simulink library "NxtrMath"  (R2013b)
settings: Solver=ode45  StartTime=0.0  StopTime=10.0  RelTol=1e-3
undefined symbols (not defined in the file or in its folder): ARCHGLBPRM_ONEOVER2PI_ULS_F32
libraries: FixdToFloat x2, FloatToFixd x2
settings Model: Creator=qzwc4r  LastModifiedBy=DZ1YRM

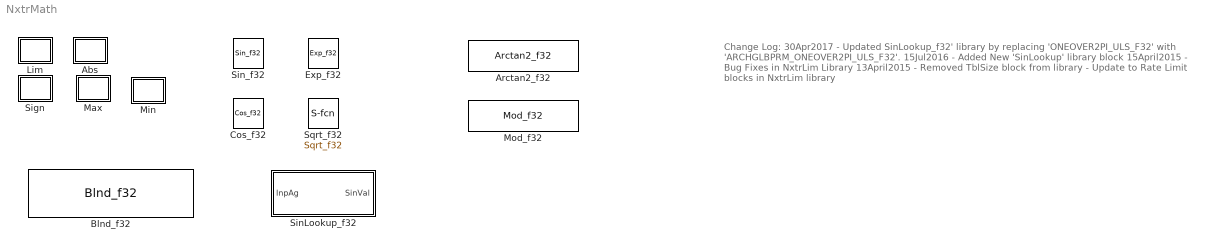
== system NxtrMath ==
  note: Change Log:
      |
      | 30Apr2017
      | - Updated SinLookup_f32' library by replacing 'ONEOVER2PI_ULS_F32' with 'ARCHGLBPRM_ONEOVER2PI_ULS_F32'.
      |
      | 15Jul2016
      | - Added New 'SinLookup' library block
      |
      |
      | 15April2015
      | - Bug Fixes in NxtrLim Library
      |
      |
      | 13April2015
      | - Removed TblSize block from library
      | - Update to Rate Limit blocks in NxtrLim library
  Abs : Subsystem
      settings: OpenFcn=NxtrAbslt
      mask Display: fprintf('|u|')
  Arctan2_f32 : S-Function  FunctionName=Arctan2_f32  EnableBusSupport=off  mask(Arctan2_f32){SFunctionSpec=single y1 = Arctan2_f32(single u1, single u2)}
      mask help:
      | This block allows you to call the legacy functions specified by the following Legacy Code Tool definition:
      | def.SFunctionName = 'Arctan2_f32';
      | def.OutputFcnSpec = 'single y1 = Arctan2_f32(single u1, single u2)';
      | def.HeaderFiles = {'NxtrMath.h', 'Std_Types.h', 'Platform_Types.h', 'Compiler.h', 'Compiler_Cfg.h'};
      | def.IncPaths = {'..\Nexteer_Utilities v3.0.0\SrcFiles'};
      settings: AttributesFormatString=%<MaskType>
      mask Help: <p>This block was generated automatically by the Legacy Code Tool. For detailed help on this tool, call<a href="matlab:legacy_code('help')"> legacy_code('help')</a>.</p>
      mask Display:
      | % time = (-0.4:0.001:0.4)
      | % plot(time+0.5,0.35*atan(20*pi*(time))+0.51)
      | fprintf('Arctan2')
      | port_label('input',1,'Numer')
      | port_label('input',2,'Denom')
      | port_label('Output',1,'Outp')
  Blnd_f32 : S-Function  FunctionName=Blnd_f32  EnableBusSupport=off  mask(Blnd_f32){SFunctionSpec=single y1 = Blnd_f32(single u1, single u2, single u3), Parameter3=on}
      mask prompts: Parameter3 "Show Figure"
      mask help:
      | This block allows you to call the legacy functions specified by the following Legacy Code Tool definition:
      | def.SFunctionName = 'Blnd_f32';
      | def.OutputFcnSpec = 'single y1 = Blnd_f32(single u1, single u2, single u3)';
      | def.HeaderFiles = {'NxtrMath.h', 'Std_Types.h', 'Platform_Types.h', 'Compiler.h', 'Compiler_Cfg.h'};
      | def.IncPaths = {'..\Nexteer_Utilities v3.0.0\SrcFiles'};
      settings: AttributesFormatString=%<Name>
      mask Help: <p>This block was generated automatically by the Legacy Code Tool. For detailed help on this tool, call<a href="matlab:legacy_code('help')"> legacy_code('help')</a>.</p>
      mask Display:
      | port_label('input',1,'Inp1')
      | port_label('input',2,'Inp2')
      | port_label('input',3,'Fac')
      | port_label('output',1,'Outp')
      | if Parameter3 == 1
      |     text(0.2,0.6,'\nInp1*(1 -Fac) ->|----|\n                        | + |-->\n    (Inp2*Fac) ->|----|')
      | end
  Cos_f32 : S-Function  FunctionName=Cos_f32  EnableBusSupport=off  mask(Cos_f32){SFunctionSpec=single y1 = Cos_f32(single u1)}
      mask help:
      | This block allows you to call the legacy functions specified by the following Legacy Code Tool definition:
      | def.SFunctionName = 'Cos_f32';
      | def.OutputFcnSpec = 'single y1 = Cos_f32(single u1)';
      | def.HeaderFiles = {'NxtrMath.h', 'Std_Types.h', 'Platform_Types.h', 'Compiler.h', 'Compiler_Cfg.h'};
      | def.IncPaths = {'..\Nexteer_Utilities v3.0.0\SrcFiles'};
      settings: AttributesFormatString=%<MaskType>
      mask Help: <p>This block was generated automatically by the Legacy Code Tool. For detailed help on this tool, call<a href="matlab:legacy_code('help')"> legacy_code('help')</a>.</p>
      mask Display: fprintf('Cos')
  Exp_f32 : S-Function  FunctionName=Exp_f32  EnableBusSupport=off  mask(Exp_f32){SFunctionSpec=single y1 = Exp_f32(single u1), ShowSpec=on}
      mask prompts: ShowSpec "Display function specification"
      mask help:
      | This block allows you to call the legacy functions specified by the following Legacy Code Tool definition:
      | def.SFunctionName = 'Exp_f32';
      | def.OutputFcnSpec = 'single y1 = Exp_f32(single u1)';
      | def.HeaderFiles = {'NxtrMath.h', 'Std_Types.h', 'Platform_Types.h', 'Compiler.h', 'Compiler_Cfg.h'};
      | def.IncPaths = {'..\Nexteer_Utilities v3.0.0\SrcFiles'};
      settings: AttributesFormatString=%<MaskType>
      mask Help: <p>This block was generated automatically by the Legacy Code Tool. For detailed help on this tool, call<a href="matlab:legacy_code('help')"> legacy_code('help')</a>.</p>
      mask Callback ShowSpec:
      | if strcmp(get_param(gcbh, 'ShowSpec'), 'on')
      |   set_param(gcbh, 'MaskDisplay', sprintf('fprintf(''%s'');', get_param(gcbh, 'SFunctionSpec')));
      | else
      |   set_param(gcbh, 'MaskDisplay', sprintf('fprintf(''%s'');', get_param(gcbh, 'FunctionName')));
      | end
      mask Display: fprintf('Exp');
  Lim : Subsystem
      settings: OpenFcn=NxtrLim
      mask Display: fprintf('Lim')
  Max : Subsystem
      settings: OpenFcn=NxtrMax
      mask Display: fprintf('Max')
  Min : Subsystem
      settings: OpenFcn=NxtrMin
      mask Display: fprintf('Min')
  Mod_f32 : S-Function  FunctionName=Mod_f32  EnableBusSupport=off  mask(Mod_f32){SFunctionSpec=single y1 = Mod_f32(single u1, single u2)}
      mask help:
      | This block allows you to call the legacy functions specified by the following Legacy Code Tool definition:
      | def.SFunctionName = 'Mod_f32';
      | def.OutputFcnSpec = 'single y1 = Mod_f32(single u1, single u2)';
      | def.HeaderFiles = {'NxtrMath.h', 'Std_Types.h', 'Platform_Types.h', 'Compiler.h', 'Compiler_Cfg.h'};
      | def.IncPaths = {'..\Nexteer_Utilities v3.0.0\SrcFiles'};
      settings: AttributesFormatString=%<MaskType>
      mask Help: <p>This block was generated automatically by the Legacy Code Tool. For detailed help on this tool, call<a href="matlab:legacy_code('help')"> legacy_code('help')</a>.</p>
      mask Display:
      | fprintf('Mod');
      | port_label('input',1,'Numer')
      | port_label('input',2,'Denom')
      | port_label('Output',1,'Outp')
  Sign : Subsystem
      settings: OpenFcn=NxtrSign
      mask Display:
      | % Xx = [-0.1, 0.1]*3;
      | % Xy = [ 0, 0];
      | % Yx = [ 0, 0];
      | % Yy = [-0.14, 0.14]*3;
      | %
      | % px = [-.1, 0, 0, 0.1]*3;
      | % py = [-.1, -.1, .1, .1]*3;
      | % plot(Xx+.5,Xy+.5, Yx+.5,Yy+.5, px+.5,py+.5)
      | fprintf('Sign')
  SinLookup_f32 : Subsystem  RequirementInfo={} %GIDa_60749778_a9c8_4d11_82e8_2a5675339b80  mask(SinLookup){}
      mask help:
      | This library block is used to calculate the Sine Value of a Input Angle based on a Lookup table.
      |
      | Input to this library block shall be in Radians and Output of this library block shall be a Unitless value.
      mask init:
      | SINCNVNCON1_ULS_F32 = single(2048);
      | SINCNVNCON2_ULS_F32 = single(1.5259021e-05);
      | SINCNVNCONTBL_ULS_U16 = uint16([0              201              402              603              804             1005             1206             1407             1608             1809             2010             2211             2412             2613             2814             3015             3216             3416             3617             3818             4019             4219             4420             4621             4821             5022             5222             5422             5623             5823             6023             6223             6424             6624             6824             7024             7223             7423             7623             7823             8022             8222             8421             8620             8820             9019             9218             9417             9616             9815            10014            10212            10411            10609            10808            11006            11204            11402            11600            11798            11996            12193            12391            12588            12785            12982            13179            13376            13573            13770            13966            14163            14359            14555            14751            14947            15142            15338            15533            15729            15924            16119            16313            16508            16703            16897            17091            17285            17479            17673            17866            18060            18253            18446            18639            18831            19024            19216            19408            19600            19792            19984            20175            20366            20557            20748            20939            21129            21319            21509            21699            21889            22078            22267            22456            22645            22834            23022            23210            23398            23586            23773            23960            24147            24334            24521            24707            24893            25079            25265            25450            25635            25820            26005            26189            26374            26557            26741            26925            27108            27291            27473            27656            27838            28020            28201            28383            28564            28745            28925            29106            29286            29465            29645            29824            30003            30181            30360            30538            30716            30893            31070            31247            31424            31600            31776            31952            32127            32302            32477            32651            32826            32999            33173            33346            33519            33692            33864            34036            34208            34379            34550            34721            34891            35061            35231            35400            35569            35738            35906            36074            36242            36409            36576            36743            36909            37075            37241            37406            37571            37736            37900            38064            38227            38390            38553            38715            38877            39039            39200            39361            39522            39682            39842            40001            40161            40319            40478            40635            40793            40950            41107            41263            41419            41575            41730            41885            42039            42194            42347            42500            42653            42806            42958            43109            43261            43411            43562            43712            43861            44011            44159            44308            44456            44603            44750            44897            45043            45189            45334            45479            45624            45768            45912            46055            46198            46340            46482            46624            46765            46905            47046            47185            47325            47464            47602            47740            47877            48014            48151            48287            48423            48558            48693            48827            48961            49095            49228            49360            49492            49624            49755            49885            50016            50145            50274            50403            50531            50659            50787            50913            51040            51166            51291            51416            51540            51664            51788            51911            52033            52155            52277            52398            52518            52638            52758            52877            52995            53113            53231            53348            53464            53580            53696            53811            53925            54039            54153            54266            54378            54490            54602            54713            54823            54933            55042            55151            55260            55367            55475            55582            55688            55794            55899            56003            56108            56211            56314            56417            56519            56620            56721            56822            56922            57021            57120            57218            57316            57413            57510            57606            57702            57797            57891            57985            58079            58171            58264            58356            58447            58537            58628            58717            58806            58895            58983            59070            59157            59243            59329            59414            59498            59582            59666            59749            59831            59913            59994            60075            60155            60234            60313            60391            60469            60546            60623            60699            60775            60850            60924            60998            61071            61144            61216            61287            61358            61429            61498            61567            61636            61704            61772            61838            61905            61970            62035            62100            62164            62227            62290            62352            62414            62475            62535            62595            62654            62713            62771            62829            62886            62942            62998            63053            63107            63161            63214            63267            63319            63371            63422            63472            63522            63571            63620            63668            63715            63762            63808            63853            63898            63943            63986            64030            64072            64114            64155            64196            64236            64276            64315            64353            64391            64428            64464            64500            64535            64570            64604            64638            64671            64703            64734            64765            64796            64826            64855            64883            64911            64939            64966            64992            65017            65042            65066            65090            65113            65136            65158            65179            65199            65219            65239            65258            65276            65293            65310            65327            65342            65357            65372            65386            65399            65412            65424            65435            65446            65456            65466            65475            65483            65491            65498            65504            65510            65515            65520            65524            65527            65530            65532            65534            65535            65535]);
      | ONEOVER2PI_ULS_F32 = single(0.1591549);
      | ONEOVER2_ULS_F32 = single(0.5);
      | ONEOVER4_ULS_F32 = single(0.25);
  Sin_f32 : S-Function  FunctionName=Sin_f32  EnableBusSupport=off  mask(Sin_f32){SFunctionSpec=single y1 = Sin_f32(single u1)}
      mask help:
      | This block allows you to call the legacy functions specified by the following Legacy Code Tool definition:
      | def.SFunctionName = 'Sin_f32';
      | def.OutputFcnSpec = 'single y1 = Sin_f32(single u1)';
      | def.HeaderFiles = {'NxtrMath.h', 'Std_Types.h', 'Platform_Types.h', 'Compiler.h', 'Compiler_Cfg.h'};
      | def.IncPaths = {'..\Nexteer_Utilities v3.0.0\SrcFiles'};
      settings: AttributesFormatString=%<MaskType>
      mask Help: <p>This block was generated automatically by the Legacy Code Tool. For detailed help on this tool, call<a href="matlab:legacy_code('help')"> legacy_code('help')</a>.</p>
      mask Display: fprintf('Sin')
  Sqrt_f32 : S-Function  FunctionName=Sqrt_f32  EnableBusSupport=off  mask(Sqrt_f32){SFunctionSpec=single y1 = Sqrt_f32(single u1), ShowSpec=on}
      mask prompts: ShowSpec "Display function specification"
      mask help:
      | This block allows you to call the legacy functions specified by the following Legacy Code Tool definition:
      | def.SFunctionName = 'Sqrt_f32';
      | def.OutputFcnSpec = 'single y1 = Sqrt_f32(single u1)';
      | def.HeaderFiles = {'NxtrMath.h', 'Std_Types.h', 'Platform_Types.h', 'Compiler.h', 'Compiler_Cfg.h'};
      | def.IncPaths = {'..\Nexteer_Utilities v3.0.0\SrcFiles'};
      settings: AttributesFormatString=%<MaskType>
      mask Help: <p>This block was generated automatically by the Legacy Code Tool. For detailed help on this tool, call<a href="matlab:legacy_code('help')"> legacy_code('help')</a>.</p>
      mask Callback ShowSpec:
      | if strcmp(get_param(gcbh, 'ShowSpec'), 'on')
      |   set_param(gcbh, 'MaskDisplay', sprintf('fprintf(''%s'');', get_param(gcbh, 'SFunctionSpec')));
      | else
      |   set_param(gcbh, 'MaskDisplay', sprintf('fprintf(''%s'');', get_param(gcbh, 'FunctionName')));
      | end
      mask Display: fprintf('single y1 = Sqrt_f32(single u1)');

== system NxtrMath/Abs ==

== system NxtrMath/Lim ==

== system NxtrMath/Max ==

== system NxtrMath/Min ==

== system NxtrMath/Sign ==

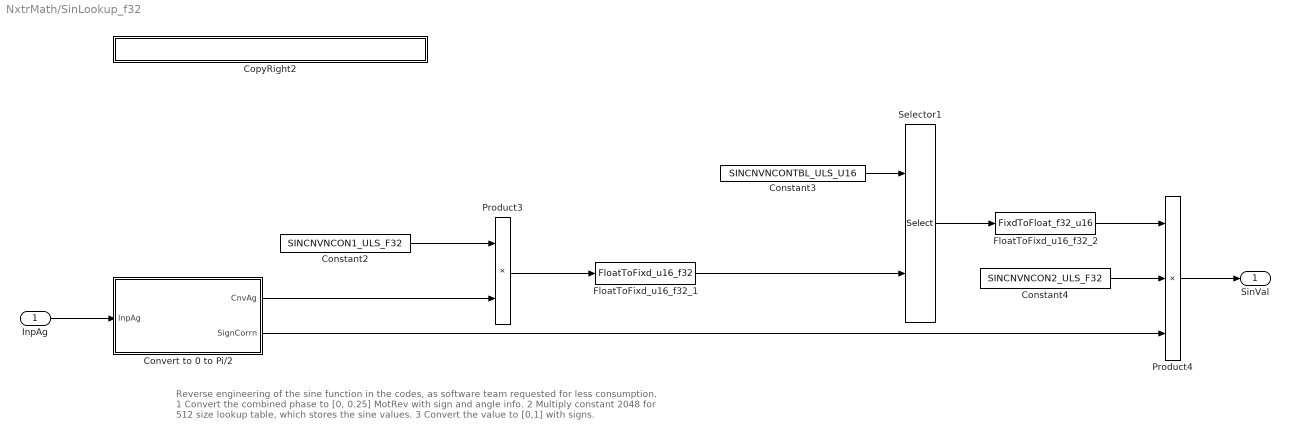
== system NxtrMath/SinLookup_f32 ==
  note: Reverse engineering of the sine function in the codes, as software team requested for less consumption.
      | 1 Convert the combined phase to [0, 0.25] MotRev with sign and angle info.
      | 2 Multiply constant 2048 for 512 size lookup table, which stores the sine values.
      | 3 Convert the value to [0,1] with signs.
  InpAg : Inport
  Constant2 : Constant  Value=SINCNVNCON1_ULS_F32
  Constant3 : Constant  Value=SINCNVNCONTBL_ULS_U16
  Constant4 : Constant  Value=SINCNVNCON2_ULS_F32
  Convert to 0 to Pi/2 : Subsystem
  CopyRight2 : Subsystem  Description=|  mask(Copyright Information){none=on}
      | Copyright info block.                                               
      |                                                                     
      | Place copyright information at the top of every subsystem in design.
      mask prompts: none "No parameters"
      mask help: Place copyright information at the top of every subsystem in design.
      mask Display:
      | NxtrConf = 'Nexteer Confidential';
      | 
      | sys = bdroot; %handle for the current model ("system")
      | first = get_param(sys,'Created');
      | if(isempty(first))
      |     first = datestr(now,'yyyy');
      | else
      |     first = first(end-3:end);  %year is last four digits
      | end
      | 
      | last = get_param(sys,'LastModifiedDate');
      | if isempty(last)
      |     last = datestr(now,'yyyy');
      | else
      |     last = last(end-3:end);
      | end
      | 
      | if strcmp(first,last)
      |     fprintf('%s -- Copyright %s Nexteer',NxtrConf,first)
      | else
      |     fprintf('%s -- %s%s- %s Nexteer',NxtrConf,char(169),first,last)
      | end
  FloatToFixd_u16_f32_1 : FloatToFixd/FloatToFixd_u16_f32  Param1=0
  FloatToFixd_u16_f32_2 : FixdToFloat/FixdToFloat_f32_u16  Param1=0
  Product3 : Product
  Product4 : Product  Inputs=3
  Selector1 : Selector  IndexMode=Zero-based  InputPortWidth=513  IndexOptions=Index vector (port)  Indices=[1 3]  OutputSizes=1
  SinVal : Outport
  wires:
  Product4/1 -> SinVal/1
  FloatToFixd_u16_f32_2/1 -> Product4/1
  Constant4/1 -> Product4/2
  Selector1/1 -> FloatToFixd_u16_f32_2/1
  Product3/1 -> FloatToFixd_u16_f32_1/1
  Constant2/1 -> Product3/1
  Constant3/1 -> Selector1/1
  InpAg/1 -> Convert to 0 to Pi/2/1(InpAg)
  Convert to 0 to Pi/2/1(CnvAg) -> Product3/2
  Convert to 0 to Pi/2/2(SignCorrn) -> Product4/3
  FloatToFixd_u16_f32_1/1 -> Selector1/2

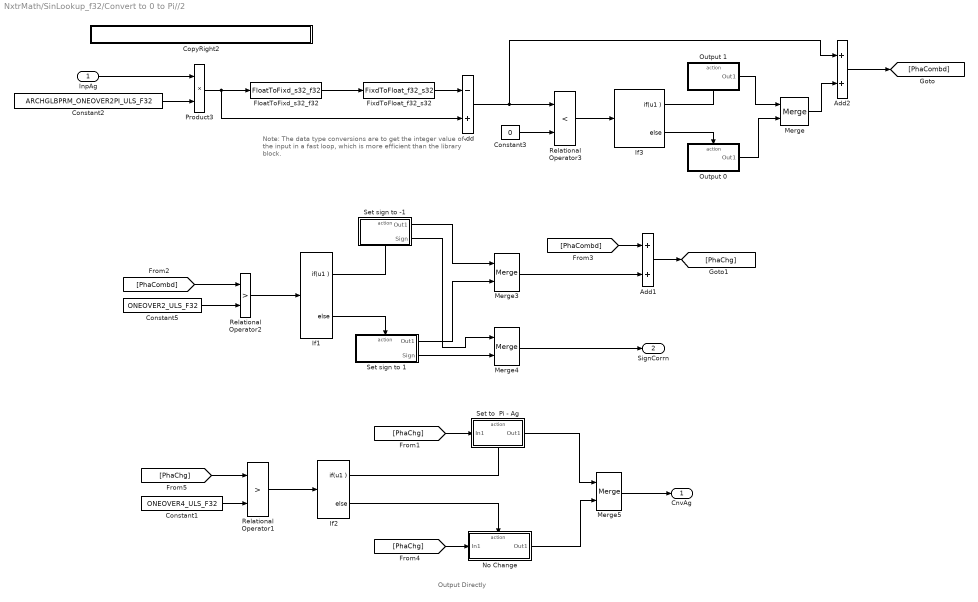
== system NxtrMath/SinLookup_f32/Convert to 0 to Pi//2 ==
  note: Note: The data type conversions are to get the integer value of
      | the input in a fast loop, which is more efficient than the library
      | block.
  note: Output Directly
  InpAg : Inport
  Add : Sum  Inputs=-+
  Add1 : Sum
  Add2 : Sum
  Constant1 : Constant  Value=ONEOVER4_ULS_F32
  Constant2 : Constant  Value=ARCHGLBPRM_ONEOVER2PI_ULS_F32
  Constant3 : Constant  Value=0  OutDataTypeStr=single
      settings: AttributesFormatString=%<OutDataTypeStr>
  Constant5 : Constant  Value=ONEOVER2_ULS_F32
  CopyRight2 : Subsystem  Description=|  mask(Copyright Information){none=on}
      | Copyright info block.                                               
      |                                                                     
      | Place copyright information at the top of every subsystem in design.
      mask prompts: none "No parameters"
      mask help: Place copyright information at the top of every subsystem in design.
      mask Display:
      | NxtrConf = 'Nexteer Confidential';
      | 
      | sys = bdroot; %handle for the current model ("system")
      | first = get_param(sys,'Created');
      | if(isempty(first))
      |     first = datestr(now,'yyyy');
      | else
      |     first = first(end-3:end);  %year is last four digits
      | end
      | 
      | last = get_param(sys,'LastModifiedDate');
      | if isempty(last)
      |     last = datestr(now,'yyyy');
      | else
      |     last = last(end-3:end);
      | end
      | 
      | if strcmp(first,last)
      |     fprintf('%s -- Copyright %s Nexteer',NxtrConf,first)
      | else
      |     fprintf('%s -- %s%s- %s Nexteer',NxtrConf,char(169),first,last)
      | end
  FixdToFloat_f32_s32 : FixdToFloat/FixdToFloat_f32_s32  Param1=0
  FloatToFixd_s32_f32 : FloatToFixd/FloatToFixd_s32_f32  Param1=0
  If1 : If  IfExpression=u1
  If2 : If  IfExpression=u1
  If3 : If  IfExpression=u1
  Merge{,3..5} (4 alike) : Merge
  No Change : Subsystem  TreatAsAtomicUnit=on
  Output 0 : Subsystem  TreatAsAtomicUnit=on
  Output 1 : Subsystem  TreatAsAtomicUnit=on
  Product3 : Product
  Relational Operator1 : RelationalOperator  Operator=>  OutDataTypeStr=boolean
  Relational Operator2 : RelationalOperator  Operator=>  OutDataTypeStr=boolean
  Relational Operator3 : RelationalOperator  Operator=<  OutDataTypeStr=boolean
  Set sign to -1 : Subsystem  TreatAsAtomicUnit=on
  Set sign to 1 : Subsystem  TreatAsAtomicUnit=on
  Set to  Pi - Ag : Subsystem  TreatAsAtomicUnit=on
  CnvAg : Outport
  SignCorrn : Outport  Port=2
  wires:
  Merge4/1 -> SignCorrn/1
  Merge5/1 -> CnvAg/1
  Set sign to 1/2(Sign) -> Merge4/2
  Relational Operator1/1 -> If2/1
  [PhaCombd] -> Relational Operator2/1
  If2/1 -> Set to  Pi - Ag/Action
  Constant5/1 -> Relational Operator2/2
  [PhaCombd] -> Add1/1
  Merge3/1 -> Add1/2
  If2/2 -> No Change/Action
  Set sign to -1/1(Out1) -> Merge3/1
  Set sign to 1/1(Out1) -> Merge3/2
  [PhaChg] -> Set to  Pi - Ag/1(In1)
  If1/1 -> Set sign to -1/Action
  No Change/1(Out1) -> Merge5/2
  Add1/1 -> [PhaChg]
  Set sign to -1/2(Sign) -> Merge4/1
  Set to  Pi - Ag/1(Out1) -> Merge5/1
  Constant1/1 -> Relational Operator1/2
  If1/2 -> Set sign to 1/Action
  Relational Operator2/1 -> If1/1
  InpAg/1 -> Product3/1
  Product3/1 -> Add/2, FloatToFixd_s32_f32/1
  Constant2/1 -> Product3/2
  [PhaChg] -> No Change/1(In1)
  [PhaChg] -> Relational Operator1/1
  FloatToFixd_s32_f32/1 -> FixdToFloat_f32_s32/1
  FixdToFloat_f32_s32/1 -> Add/1
  Add/1 -> Add2/1, Relational Operator3/1
  Relational Operator3/1 -> If3/1
  Constant3/1 -> Relational Operator3/2
  If3/1 -> Output 1/Action
  If3/2 -> Output 0/Action
  Output 1/1(Out1) -> Merge/1
  Output 0/1(Out1) -> Merge/2
  Add2/1 -> [PhaCombd]
  Merge/1 -> Add2/2

== system NxtrMath/SinLookup_f32/CopyRight2 ==

== system NxtrMath/SinLookup_f32/Convert to 0 to Pi//2/CopyRight2 ==

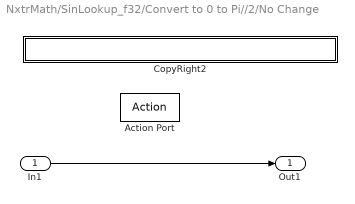
== system NxtrMath/SinLookup_f32/Convert to 0 to Pi//2/No Change ==
  In1 : Inport
  Action Port : ActionPort
  CopyRight2 : Subsystem  Description=|  mask(Copyright Information){none=on}
      | Copyright info block.                                               
      |                                                                     
      | Place copyright information at the top of every subsystem in design.
      mask prompts: none "No parameters"
      mask help: Place copyright information at the top of every subsystem in design.
      mask Display:
      | NxtrConf = 'Nexteer Confidential';
      | 
      | sys = bdroot; %handle for the current model ("system")
      | first = get_param(sys,'Created');
      | if(isempty(first))
      |     first = datestr(now,'yyyy');
      | else
      |     first = first(end-3:end);  %year is last four digits
      | end
      | 
      | last = get_param(sys,'LastModifiedDate');
      | if isempty(last)
      |     last = datestr(now,'yyyy');
      | else
      |     last = last(end-3:end);
      | end
      | 
      | if strcmp(first,last)
      |     fprintf('%s -- Copyright %s Nexteer',NxtrConf,first)
      | else
      |     fprintf('%s -- %s%s- %s Nexteer',NxtrConf,char(169),first,last)
      | end
  Out1 : Outport
  wires:
  In1/1 -> Out1/1

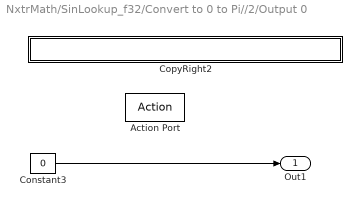
== system NxtrMath/SinLookup_f32/Convert to 0 to Pi//2/Output 0 ==
  Action Port : ActionPort
  Constant3 : Constant  Value=0  OutDataTypeStr=single
      settings: AttributesFormatString=%<OutDataTypeStr>
  CopyRight2 : Subsystem  Description=|  mask(Copyright Information){none=on}
      | Copyright info block.                                               
      |                                                                     
      | Place copyright information at the top of every subsystem in design.
      mask prompts: none "No parameters"
      mask help: Place copyright information at the top of every subsystem in design.
      mask Display:
      | NxtrConf = 'Nexteer Confidential';
      | 
      | sys = bdroot; %handle for the current model ("system")
      | first = get_param(sys,'Created');
      | if(isempty(first))
      |     first = datestr(now,'yyyy');
      | else
      |     first = first(end-3:end);  %year is last four digits
      | end
      | 
      | last = get_param(sys,'LastModifiedDate');
      | if isempty(last)
      |     last = datestr(now,'yyyy');
      | else
      |     last = last(end-3:end);
      | end
      | 
      | if strcmp(first,last)
      |     fprintf('%s -- Copyright %s Nexteer',NxtrConf,first)
      | else
      |     fprintf('%s -- %s%s- %s Nexteer',NxtrConf,char(169),first,last)
      | end
  Out1 : Outport
  wires:
  Constant3/1 -> Out1/1

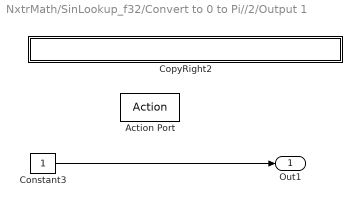
== system NxtrMath/SinLookup_f32/Convert to 0 to Pi//2/Output 1 ==
  Action Port : ActionPort
  Constant3 : Constant  OutDataTypeStr=single
      settings: AttributesFormatString=%<OutDataTypeStr>
  CopyRight2 : Subsystem  Description=|  mask(Copyright Information){none=on}
      | Copyright info block.                                               
      |                                                                     
      | Place copyright information at the top of every subsystem in design.
      mask prompts: none "No parameters"
      mask help: Place copyright information at the top of every subsystem in design.
      mask Display:
      | NxtrConf = 'Nexteer Confidential';
      | 
      | sys = bdroot; %handle for the current model ("system")
      | first = get_param(sys,'Created');
      | if(isempty(first))
      |     first = datestr(now,'yyyy');
      | else
      |     first = first(end-3:end);  %year is last four digits
      | end
      | 
      | last = get_param(sys,'LastModifiedDate');
      | if isempty(last)
      |     last = datestr(now,'yyyy');
      | else
      |     last = last(end-3:end);
      | end
      | 
      | if strcmp(first,last)
      |     fprintf('%s -- Copyright %s Nexteer',NxtrConf,first)
      | else
      |     fprintf('%s -- %s%s- %s Nexteer',NxtrConf,char(169),first,last)
      | end
  Out1 : Outport
  wires:
  Constant3/1 -> Out1/1

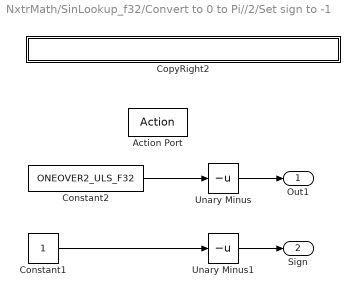
== system NxtrMath/SinLookup_f32/Convert to 0 to Pi//2/Set sign to -1 ==
  Action Port : ActionPort
  Constant1 : Constant  OutDataTypeStr=single
      settings: AttributesFormatString=%<OutDataTypeStr>
  Constant2 : Constant  Value=ONEOVER2_ULS_F32
  CopyRight2 : Subsystem  Description=|  mask(Copyright Information){none=on}
      | Copyright info block.                                               
      |                                                                     
      | Place copyright information at the top of every subsystem in design.
      mask prompts: none "No parameters"
      mask help: Place copyright information at the top of every subsystem in design.
      mask Display:
      | NxtrConf = 'Nexteer Confidential';
      | 
      | sys = bdroot; %handle for the current model ("system")
      | first = get_param(sys,'Created');
      | if(isempty(first))
      |     first = datestr(now,'yyyy');
      | else
      |     first = first(end-3:end);  %year is last four digits
      | end
      | 
      | last = get_param(sys,'LastModifiedDate');
      | if isempty(last)
      |     last = datestr(now,'yyyy');
      | else
      |     last = last(end-3:end);
      | end
      | 
      | if strcmp(first,last)
      |     fprintf('%s -- Copyright %s Nexteer',NxtrConf,first)
      | else
      |     fprintf('%s -- %s%s- %s Nexteer',NxtrConf,char(169),first,last)
      | end
  Unary Minus : UnaryMinus
  Unary Minus1 : UnaryMinus
  Out1 : Outport
  Sign : Outport  Port=2
  wires:
  Constant1/1 -> Unary Minus1/1
  Constant2/1 -> Unary Minus/1
  Unary Minus/1 -> Out1/1
  Unary Minus1/1 -> Sign/1

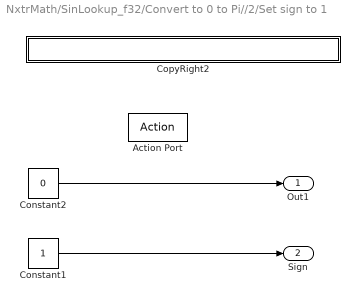
== system NxtrMath/SinLookup_f32/Convert to 0 to Pi//2/Set sign to 1 ==
  Action Port : ActionPort
  Constant1 : Constant  OutDataTypeStr=single
      settings: AttributesFormatString=%<OutDataTypeStr>
  Constant2 : Constant  Value=0  OutDataTypeStr=single
      settings: AttributesFormatString=%<OutDataTypeStr>
  CopyRight2 : Subsystem  Description=|  mask(Copyright Information){none=on}
      | Copyright info block.                                               
      |                                                                     
      | Place copyright information at the top of every subsystem in design.
      mask prompts: none "No parameters"
      mask help: Place copyright information at the top of every subsystem in design.
      mask Display:
      | NxtrConf = 'Nexteer Confidential';
      | 
      | sys = bdroot; %handle for the current model ("system")
      | first = get_param(sys,'Created');
      | if(isempty(first))
      |     first = datestr(now,'yyyy');
      | else
      |     first = first(end-3:end);  %year is last four digits
      | end
      | 
      | last = get_param(sys,'LastModifiedDate');
      | if isempty(last)
      |     last = datestr(now,'yyyy');
      | else
      |     last = last(end-3:end);
      | end
      | 
      | if strcmp(first,last)
      |     fprintf('%s -- Copyright %s Nexteer',NxtrConf,first)
      | else
      |     fprintf('%s -- %s%s- %s Nexteer',NxtrConf,char(169),first,last)
      | end
  Out1 : Outport
  Sign : Outport  Port=2
  wires:
  Constant2/1 -> Out1/1
  Constant1/1 -> Sign/1

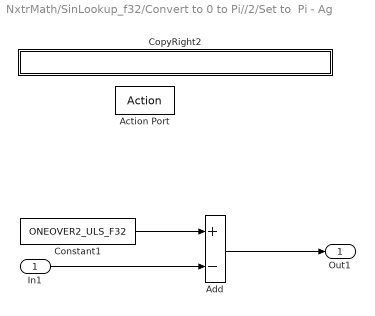
== system NxtrMath/SinLookup_f32/Convert to 0 to Pi//2/Set to  Pi - Ag ==
  In1 : Inport
  Action Port : ActionPort
  Add : Sum  Inputs=+-
  Constant1 : Constant  Value=ONEOVER2_ULS_F32
  CopyRight2 : Subsystem  Description=|  mask(Copyright Information){none=on}
      | Copyright info block.                                               
      |                                                                     
      | Place copyright information at the top of every subsystem in design.
      mask prompts: none "No parameters"
      mask help: Place copyright information at the top of every subsystem in design.
      mask Display:
      | NxtrConf = 'Nexteer Confidential';
      | 
      | sys = bdroot; %handle for the current model ("system")
      | first = get_param(sys,'Created');
      | if(isempty(first))
      |     first = datestr(now,'yyyy');
      | else
      |     first = first(end-3:end);  %year is last four digits
      | end
      | 
      | last = get_param(sys,'LastModifiedDate');
      | if isempty(last)
      |     last = datestr(now,'yyyy');
      | else
      |     last = last(end-3:end);
      | end
      | 
      | if strcmp(first,last)
      |     fprintf('%s -- Copyright %s Nexteer',NxtrConf,first)
      | else
      |     fprintf('%s -- %s%s- %s Nexteer',NxtrConf,char(169),first,last)
      | end
  Out1 : Outport
  wires:
  Add/1 -> Out1/1
  Constant1/1 -> Add/1
  In1/1 -> Add/2

== system NxtrMath/SinLookup_f32/Convert to 0 to Pi//2/No Change/CopyRight2 ==

== system NxtrMath/SinLookup_f32/Convert to 0 to Pi//2/Output 0/CopyRight2 ==

== system NxtrMath/SinLookup_f32/Convert to 0 to Pi//2/Output 1/CopyRight2 ==

== system NxtrMath/SinLookup_f32/Convert to 0 to Pi//2/Set sign to -1/CopyRight2 ==

== system NxtrMath/SinLookup_f32/Convert to 0 to Pi//2/Set sign to 1/CopyRight2 ==

== system NxtrMath/SinLookup_f32/Convert to 0 to Pi//2/Set to  Pi - Ag/CopyRight2 ==
